simulink model "SVPWM_STM32_Sim"  (R2026a)
settings: Solver=VariableStepAuto  StopTime=0.05
libraries: simulink x1
settings Model: Creator=lagsshin  LastModifiedBy=lagsshin

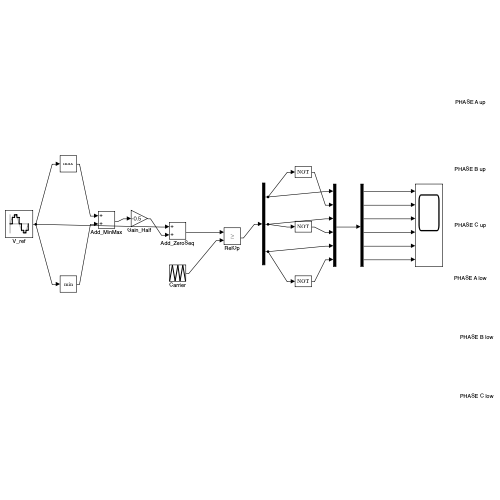
[thumbnail: Simulink's stored preview of the top-level diagram]
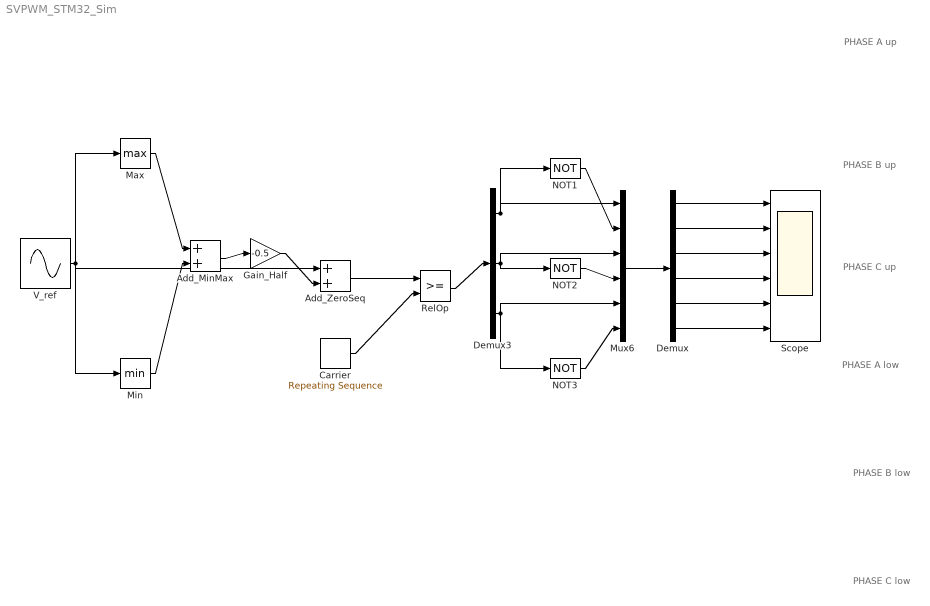
== system SVPWM_STM32_Sim ==
  note: PHASE A up
  note: PHASE B up
  note: PHASE C up
  note: PHASE A low
  note: PHASE B low
  note: PHASE C low
  Add_MinMax : Sum
  Add_ZeroSeq : Sum
  Carrier : simulink/Sources/Repeating Sequence  rep_seq_t=[0, 25e-6, 50e-6]  rep_seq_y=[-1, 1, -1]
  Demux : Demux  Outputs=6
  Demux3 : Demux  Outputs=3
  Gain_Half : Gain  Gain=-0.5
  Max : MinMax  Function=max
  Min : MinMax
  Mux6 : Mux  Inputs=6
  NOT1 : Logic  Operator=NOT  AllPortsSameDT=off  OutDataTypeStr=boolean
  NOT2 : Logic  Operator=NOT  AllPortsSameDT=off  OutDataTypeStr=boolean
  NOT3 : Logic  Operator=NOT  AllPortsSameDT=off  OutDataTypeStr=boolean
  RelOp : RelationalOperator  OutDataTypeStr=boolean  RndMeth=Simplest  InputSameDT=off
  Scope : Scope  NumInputPorts=6
      settings: ActiveDisplayYMinimum=0.60935533631397232  ActiveDisplayYMaximum=0.76537499847405221
  V_ref : Sin  Amplitude=0.8  Frequency=50*2*pi  Phase=[0, -2*pi/3, 2*pi/3]  SampleTime=1e-6
  wires:
  V_ref/1 -> Max/1, Min/1, Add_ZeroSeq/1
  Max/1 -> Add_MinMax/1
  Min/1 -> Add_MinMax/2
  Add_MinMax/1 -> Gain_Half/1
  Gain_Half/1 -> Add_ZeroSeq/2
  Add_ZeroSeq/1 -> RelOp/1
  Carrier/1 -> RelOp/2
  RelOp/1 -> Demux3/1
  Demux3/1 -> NOT1/1, Mux6/1
  Demux3/2 -> NOT2/1, Mux6/3
  Demux3/3 -> NOT3/1, Mux6/5
  NOT1/1 -> Mux6/2
  NOT2/1 -> Mux6/4
  NOT3/1 -> Mux6/6
  Mux6/1 -> Demux/1
  Demux/1 -> Scope/1
  Demux/2 -> Scope/2
  Demux/3 -> Scope/3
  Demux/4 -> Scope/4
  Demux/5 -> Scope/5
  Demux/6 -> Scope/6
